simulink model "NPC_1"  (R2013a)
settings: Solver=FixedStepDiscrete  SolverMode=SingleTasking  StartTime=0.0  StopTime=1  FixedStep=Ts  MaxStep=100e-6  MinStep=50e-6  RelTol=1e-3
InitFcn:
  | Ts = 1e-6
libraries: powerlib x72, simulink x6, powerlib_meascontrol x3
settings Model: Creator=Daniel  LastModifiedBy=Daniel
settings SolverCC: InitialStep=50e-6  MaxConsecutiveMinStep=100000  AlgebraicLoopSolver=LineSearch
settings DebuggingCC: ArrayBoundsChecking=warning  AlgebraicLoopMsg=none  ArtificialAlgebraicLoopMsg=none  ParameterPrecisionLossMsg=none  UnconnectedInputMsg=none  UnconnectedOutputMsg=none  UnconnectedLineMsg=none

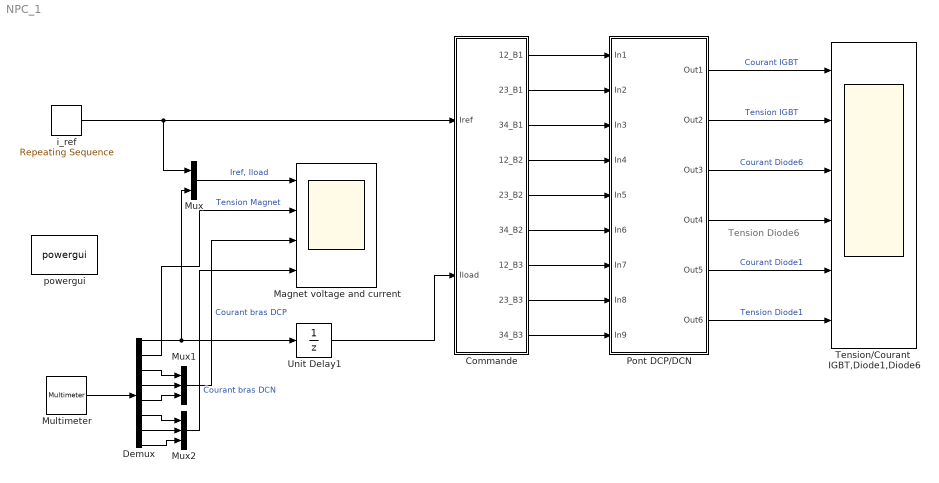
== system NPC_1 ==
  note: Tension Diode6
  Commande : Subsystem  SystemSampleTime=Ts
      settings: MinAlgLoopOccurrences=on
  Demux : Demux  Outputs=8
  Magnet voltage and current : Scope  NumInputPorts=4
      settings: YMin=970~-1000~-12500~-12500  YMax=1030~5000~12500~12500
  Multimeter : powerlib/Measurements/Multimeter  PhasorSimulation=off  OutputType=Complex  sel=[2 1 3 4 5 6 7 8]  L=8  Gain=[1 1 1 1 1 1 1 1]  yselected={'Ib: Pont DCP//DCN/Magnet','Ub: Pont DCP//DCN/Magnet','Ib: Pont DCP//DCN/DC2_B1','Ib: Pont DCP//DCN/DC1_B1','Ib: Pont DCP//DCN/DC1_B2','Ib: Pont DCP//DCN/DC1_B3','Ib: Pont DCP//DCN/DC2_B2','Ib: Pont DCP//DCN/DC2_B3'};  PSBOutputType=1  PSBequivalent=0  AxesSetting=[0,0.1,-100,100]  Display=0  SavedBlockNames=-11
  Mux : Mux  Inputs=2
  Mux1 : Mux  Inputs=3
  Mux2 : Mux  Inputs=3
  Pont DCP/DCN : Subsystem  SystemSampleTime=Ts
      settings: MinAlgLoopOccurrences=on
  Tension/Courant  IGBT,Diode1,Diode6 : Scope  NumInputPorts=6
      settings: YMin=0~-500~0~-2500~-1~-2750  YMax=17500~2500~2000~500~1~0  SaveName=ScopeData2
  Unit Delay1 : UnitDelay  SampleTime=-1
  "i_ref " : simulink/Sources/Repeating Sequence  rep_seq_t=[0 100e-3 475e-3 550e-3 675e-3 900e-3]  rep_seq_y=[0 250 6000 6000 250 250]
  powergui : powerlib/powergui  Priority=1  SimulationMode=Discrete  SolverType=Tustin  SampleTime=Ts  frequency=60  SPID=off  DisableSnubberDevices=off  DisableRonSwitches=off  DisableVfSwitches=off  SwTol=0  Interpol=off  DisplayEquations=off  frequencyindice=0  Pbase=100e6  ErrMax=1e-4  Iterations=50  UnitsV=kV  UnitsW=MW  FunctionMessages=off  echomessages=off  HookPort=off  EnableUseOfTLC=off  x0status=blocks  RestoreLinks=warning  ResistiveCurrentMeasurement=off  Frange=[0:2:500]  Ylog=off  Xlog=on  ShowGrid=off  save=off  variable=ZData  ZoomFFT=off  StartTime=0.0  cycles=1  DisplayStyle=1  fundamental=60  FreqAxis=off  MaxFrequency=1000  frequencyindicesteady=1  RmsSteady=1  display=off  Ts=0  methode=off
  wires:
  Mux/1 -> Magnet voltage and current/1  "Iref, Iload"
  Multimeter/1 -> Demux/1
  Demux/1 -> Unit Delay1/1, Mux/2
  Demux/2 -> Magnet voltage and current/2  "Tension Magnet"
  Demux/3 -> Mux1/1
  Demux/4 -> Mux1/2
  Demux/5 -> Mux1/3
  Demux/6 -> Mux2/1
  Demux/7 -> Mux2/2
  Demux/8 -> Mux2/3
  Mux1/1 -> Magnet voltage and current/3  "Courant bras DCP"
  Mux2/1 -> Magnet voltage and current/4  "Courant bras DCN"
  Pont DCP/DCN/1(Out1) -> Tension/Courant  IGBT,Diode1,Diode6/1  "Courant IGBT"
  Pont DCP/DCN/2(Out2) -> Tension/Courant  IGBT,Diode1,Diode6/2  "Tension IGBT"
  Pont DCP/DCN/3(Out3) -> Tension/Courant  IGBT,Diode1,Diode6/3  "Courant Diode6"
  Pont DCP/DCN/4(Out4) -> Tension/Courant  IGBT,Diode1,Diode6/4
  Pont DCP/DCN/5(Out5) -> Tension/Courant  IGBT,Diode1,Diode6/5  "Courant Diode1"
  Pont DCP/DCN/6(Out6) -> Tension/Courant  IGBT,Diode1,Diode6/6  "Tension Diode1"
  Commande/1(12_B1) -> Pont DCP/DCN/1(In1)
  Commande/2(23_B1) -> Pont DCP/DCN/2(In2)
  Commande/3(34_B1) -> Pont DCP/DCN/3(In3)
  Commande/4(12_B2) -> Pont DCP/DCN/4(In4)
  Commande/5(23_B2) -> Pont DCP/DCN/5(In5)
  Commande/6("34_B2 ") -> Pont DCP/DCN/6(In6)
  Commande/7(12_B3) -> Pont DCP/DCN/7(In7)
  Commande/8(23_B3) -> Pont DCP/DCN/8(In8)
  Commande/9("34_B3 ") -> Pont DCP/DCN/9(In9)
  "i_ref "/1 -> Commande/1(Iref), Mux/1
  Unit Delay1/1 -> Commande/2("Iload ")

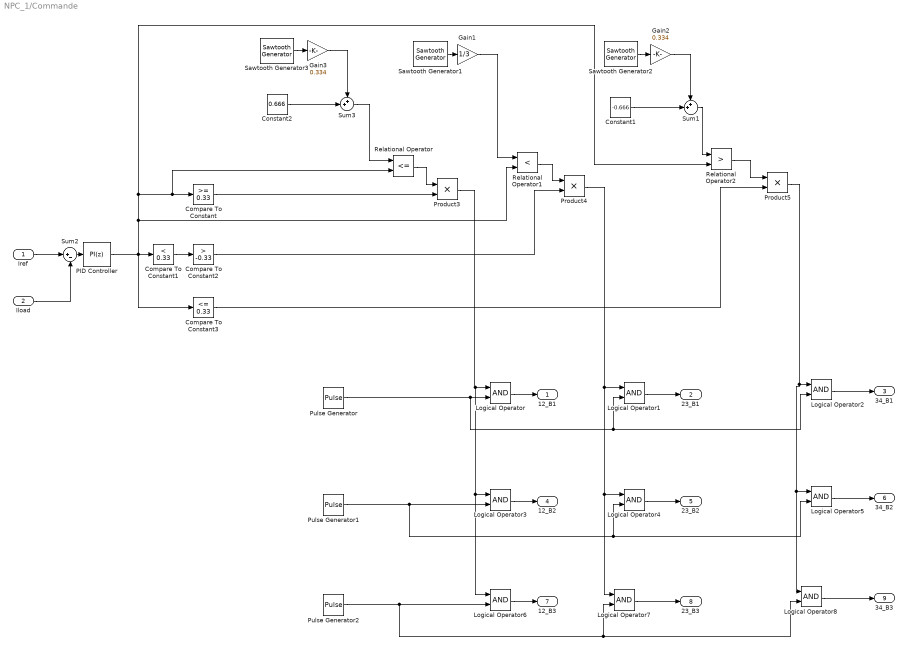
== system NPC_1/Commande ==
  Iref : Inport
  "Iload " : Inport  Port=2
  Compare To Constant : simulink/Logic and Bit Operations/Compare To Constant  relop=>=  const=0.33  OutDataTypeStr=boolean
  Compare To Constant1 : simulink/Logic and Bit Operations/Compare To Constant  relop=<  const=0.33  OutDataTypeStr=boolean
  Compare To Constant2 : simulink/Logic and Bit Operations/Compare To Constant  relop=>  const=-0.33  OutDataTypeStr=boolean
  Compare To Constant3 : simulink/Logic and Bit Operations/Compare To Constant  relop=<=  const=0.33  OutDataTypeStr=boolean
  Constant1 : Constant  Value=-0.666  SampleTime=Ts
  Constant2 : Constant  Value=0.666  SampleTime=Ts
  Gain1 : Gain  Gain=1/3  SampleTime=Ts
  Gain2 : Gain  Gain=0.334  SampleTime=Ts
  Gain3 : Gain  Gain=0.334  SampleTime=Ts
  Logical Operator{,1..8} (9 alike) : Logic  AllPortsSameDT=off  OutDataTypeStr=boolean  SampleTime=Ts
  PID Controller : simulink/Continuous/PID Controller  Controller=PI  TimeDomain=Discrete-time  SampleTime=Ts  IntegratorMethod=Forward Euler  FilterMethod=Forward Euler  Form=Parallel  P=1.05611  I=24.6  D=0  N=100  InitialConditionSource=internal  InitialConditionForIntegrator=0  InitialConditionForFilter=0  ExternalReset=none  LimitOutput=on  UpperSaturationLimit=1  LowerSaturationLimit=-1  LinearizeAsGain=on  AntiWindupMode=clamping  Kb=1  TrackingMode=off  Kt=1  PParamMin=[]  PParamMax=[]  IParamMin=[]  IParamMax=[]  DParamMin=[]  DParamMax=[]  NParamMin=[]  NParamMax=[]  KbParamMin=[]  KbParamMax=[]  KtParamMin=[]  KtParamMax=[]  POutMin=[]  POutMax=[]  IOutMin=[]  IOutMax=[]  DOutMin=[]  DOutMax=[]  NOutMin=[]  NOutMax=[]  KbOutMin=[]  KbOutMax=[]  KtOutMin=[]  KtOutMax=[]  IntegratorOutMin=[]  IntegratorOutMax=[]  FilterOutMin=[]  FilterOutMax=[]  SumOutMin=[]  SumOutMax=[]  SumI1OutMin=[]  SumI1OutMax=[]  SumI2OutMin=[]  SumI2OutMax=[]  SumI3OutMin=[]  SumI3OutMax=[]  SumDOutMin=[]  SumDOutMax=[]  SaturationOutMin=[]  SaturationOutMax=[]  IntegratorContinuousStateAttributes=''  IntegratorStateMustResolveToSignalObject=off  IntegratorRTWStateStorageClass=Auto  FilterContinuousStateAttributes=''  FilterStateMustResolveToSignalObject=off  FilterRTWStateStorageClass=Auto
  Product3 : Product  SampleTime=Ts
  Product4 : Product  SampleTime=Ts
  Product5 : Product  SampleTime=Ts
  Pulse Generator : DiscretePulseGenerator  Period=floor(3e-3/Ts)  PulseWidth=floor(1e-3/Ts)  SampleTime=Ts
  Pulse Generator1 : DiscretePulseGenerator  Period=floor(3e-3/Ts)  PulseWidth=floor(1e-3/Ts)  PhaseDelay=floor(1e-3/Ts)  SampleTime=Ts
  Pulse Generator2 : DiscretePulseGenerator  Period=floor(3e-3/Ts)  PulseWidth=floor(1e-3/Ts)  PhaseDelay=floor(2e-3/Ts)  SampleTime=Ts
  Relational Operator : RelationalOperator  Operator=<=  OutDataTypeStr=boolean  SampleTime=Ts
  Relational Operator1 : RelationalOperator  Operator=<  OutDataTypeStr=boolean  SampleTime=Ts
  Relational Operator2 : RelationalOperator  Operator=>  OutDataTypeStr=boolean  SampleTime=Ts
  Sawtooth Generator1 : powerlib_meascontrol/Pulse & Signal Generators/Sawtooth Generator  Freq=1e3  Phase=0  Ts=Ts
  Sawtooth Generator2 : powerlib_meascontrol/Pulse & Signal Generators/Sawtooth Generator  Freq=1e3  Phase=0  Ts=Ts
  Sawtooth Generator3 : powerlib_meascontrol/Pulse & Signal Generators/Sawtooth Generator  Freq=1e3  Phase=0  Ts=Ts
  Sum1 : Sum  Inputs=++|
  Sum2 : Sum  Inputs=|+-
  Sum3 : Sum  Inputs=++|
  12_B1 : Outport
  23_B1 : Outport  Port=2
  34_B1 : Outport  Port=3
  12_B2 : Outport  Port=4
  23_B2 : Outport  Port=5
  "34_B2 " : Outport  Port=6
  12_B3 : Outport  Port=7
  23_B3 : Outport  Port=8
  "34_B3 " : Outport  Port=9
  wires:
  Constant1/1 -> Sum1/2
  Sawtooth Generator1/1 -> Gain1/1
  Gain2/1 -> Sum1/1
  Sawtooth Generator2/1 -> Gain2/1
  Iref/1 -> Sum2/1
  "Iload "/1 -> Sum2/2
  Sum2/1 -> PID Controller/1
  Compare To Constant1/1 -> Compare To Constant2/1
  Compare To Constant/1 -> Product3/2
  Compare To Constant2/1 -> Product4/2
  Compare To Constant3/1 -> Product5/2
  PID Controller/1 -> Relational Operator2/2, Relational Operator/2, Compare To Constant/1, Relational Operator1/2, Compare To Constant3/1, Compare To Constant1/1
  Gain1/1 -> Relational Operator1/1
  Sum1/1 -> Relational Operator2/1
  Pulse Generator/1 -> Logical Operator2/2, Logical Operator1/2, Logical Operator/2
  Pulse Generator1/1 -> Logical Operator3/2, Logical Operator5/2, Logical Operator4/2
  Pulse Generator2/1 -> Logical Operator8/2, Logical Operator7/2, Logical Operator6/2
  Logical Operator/1 -> 12_B1/1
  Logical Operator1/1 -> 23_B1/1
  Logical Operator2/1 -> 34_B1/1
  Logical Operator4/1 -> 23_B2/1
  Logical Operator7/1 -> 23_B3/1
  Logical Operator3/1 -> 12_B2/1
  Logical Operator6/1 -> 12_B3/1
  Logical Operator5/1 -> "34_B2 "/1
  Logical Operator8/1 -> "34_B3 "/1
  Sum3/1 -> Relational Operator/1
  Relational Operator/1 -> Product3/1
  Product3/1 -> Logical Operator6/1, Logical Operator3/1, Logical Operator/1
  Relational Operator1/1 -> Product4/1
  Product4/1 -> Logical Operator7/1, Logical Operator4/1, Logical Operator1/1
  Relational Operator2/1 -> Product5/1
  Product5/1 -> Logical Operator8/1, Logical Operator5/1, Logical Operator2/1
  Constant2/1 -> Sum3/2
  Gain3/1 -> Sum3/1
  Sawtooth Generator3/1 -> Gain3/1

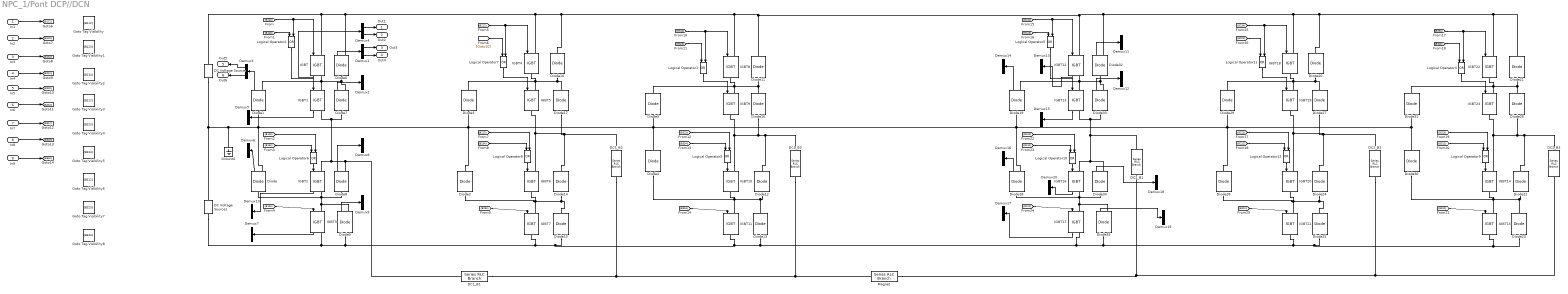
== system NPC_1/Pont DCP//DCN ==
  In1 : Inport
  In2 : Inport  Port=2
  In3 : Inport  Port=3
  In4 : Inport  Port=4
  In5 : Inport  Port=5
  In6 : Inport  Port=6
  In7 : Inport  Port=7
  In8 : Inport  Port=8
  In9 : Inport  Port=9
  DC Voltage Source : powerlib/Electrical Sources/DC Voltage Source  Amplitude=2500  Measurements=None
  DC Voltage Source1 : powerlib/Electrical Sources/DC Voltage Source  Amplitude=2500  Measurements=None
  DC1_B1 : powerlib/Elements/Series RLC Branch  LConnTagsString=__new0  RConnTagsString=__new0  BranchType=L  Resistance=0  Inductance=1e-6  SetiL0=off  InitialCurrent=0  Capacitance=1e-6  Setx0=off  InitialVoltage=0  Measurements=Branch current
  DC1_B2 : powerlib/Elements/Series RLC Branch  LConnTagsString=__new0  RConnTagsString=__new0  BranchType=L  Resistance=0  Inductance=1e-6  SetiL0=off  InitialCurrent=0  Capacitance=1e-6  Setx0=off  InitialVoltage=0  Measurements=Branch current
  DC1_B3 : powerlib/Elements/Series RLC Branch  LConnTagsString=__new0  RConnTagsString=__new0  BranchType=L  Resistance=0  Inductance=1e-6  SetiL0=off  InitialCurrent=0  Capacitance=1e-6  Setx0=off  InitialVoltage=0  Measurements=Branch current
  DC2_B1 : powerlib/Elements/Series RLC Branch  LConnTagsString=__new0  RConnTagsString=__new0  BranchType=L  Resistance=0  Inductance=1e-6  SetiL0=off  InitialCurrent=0  Capacitance=1e-6  Setx0=off  InitialVoltage=0  Measurements=Branch current
  DC2_B2 : powerlib/Elements/Series RLC Branch  LConnTagsString=__new0  RConnTagsString=__new0  BranchType=L  Resistance=0  Inductance=1e-6  SetiL0=off  InitialCurrent=0  Capacitance=1e-6  Setx0=off  InitialVoltage=0  Measurements=Branch current
  DC2_B3 : powerlib/Elements/Series RLC Branch  LConnTagsString=__new0  RConnTagsString=__new0  BranchType=L  Resistance=0  Inductance=1e-6  SetiL0=off  InitialCurrent=0  Capacitance=1e-6  Setx0=off  InitialVoltage=0  Measurements=Branch current
  Demux{1..20} (20 alike) : Demux  Outputs=2
  Diode{,1,6..9,18..19,32..35} (12 alike) : powerlib/Power Electronics/Diode  Ron=0.001  Lon=0  Vf=0.8  IC=0  UseSnubber=off  Rs=1  Cs=inf  Measurements=on
  Diode{2..5,10..17,20..31} (24 alike) : powerlib/Power Electronics/Diode  Ron=0.001  Lon=0  Vf=0.8  IC=0  UseSnubber=off  Rs=1  Cs=inf  Measurements=off
  Goto Tag Visibility : GotoTagVisibility  GotoTag=B112
  Goto Tag Visibility1 : GotoTagVisibility  GotoTag=B123
  Goto Tag Visibility2 : GotoTagVisibility  GotoTag=B134
  Goto Tag Visibility3 : GotoTagVisibility  GotoTag=B212
  Goto Tag Visibility4 : GotoTagVisibility  GotoTag=B223
  Goto Tag Visibility5 : GotoTagVisibility  GotoTag=B234
  Goto Tag Visibility6 : GotoTagVisibility  GotoTag=B312
  Goto Tag Visibility7 : GotoTagVisibility  GotoTag=B323
  Goto Tag Visibility8 : GotoTagVisibility  GotoTag=B334
  Ground2 : powerlib/Elements/Ground  LConnTagsString=a
  IGBT{,1..3,12..13,16..17} (8 alike) : powerlib/Power Electronics/IGBT  Ron=0.001  Lon=0  Vf=1  Tf=1e-6  Tt=2e-6  IC=0  Rs=0  Cs=0  Measurements=on
  IGBT{4..11,14..15,18..23} (16 alike) : powerlib/Power Electronics/IGBT  Ron=0.001  Lon=0  Vf=1  Tf=1e-6  Tt=2e-6  IC=0  Rs=0  Cs=0  Measurements=off
  Logical Operator{1..12} (12 alike) : Logic  Operator=OR  AllPortsSameDT=off  OutDataTypeStr=boolean
  Magnet : powerlib/Elements/Series RLC Branch  LConnTagsString=__new0  RConnTagsString=__new0  BranchType=RL  Resistance=0.28  Inductance=0.1  SetiL0=off  InitialCurrent=0  Capacitance=1e-6  Setx0=off  InitialVoltage=0  Measurements=Branch voltage and current
  Out1 : Outport
  Out2 : Outport  Port=2
  Out3 : Outport  Port=3
  Out4 : Outport  Port=4
  Out5 : Outport  Port=5
  Out6 : Outport  Port=6
  tag scope: B112=scoped, B123=scoped, B134=scoped, B212=scoped, B223=scoped, B234=scoped, B312=scoped, B323=scoped, B334=scoped
  wires:
  IGBT12/1 -> Demux13/1
  Diode34/1 -> Demux18/1
  Diode35/1 -> Demux19/1
  Logical Operator7/1 -> IGBT5/1
  Diode7/1 -> Demux2/1
  Logical Operator3/1 -> IGBT10/1
  Logical Operator1/1 -> IGBT9/1
  [B323] -> Logical Operator3/2
  [B334] -> Logical Operator3/1
  [B123] -> Logical Operator10/2
  Diode18/1 -> Demux16/1
  Logical Operator10/1 -> IGBT16/1
  [B223] -> Logical Operator12/2
  [B112] -> IGBT17/1
  [B212] -> IGBT21/1
  [B123] -> Logical Operator5/1
  [B112] -> Logical Operator10/1
  [B212] -> Logical Operator12/1
  Logical Operator6/1 -> IGBT2/1
  [B223] -> Logical Operator8/2
  [B112] -> IGBT/1, Logical Operator2/2
  [B323] -> Logical Operator1/1
  [B234] -> Logical Operator8/1
  Diode1/1 -> Demux3/1
  [B234] -> Logical Operator11/2, IGBT18/1
  [B334] -> IGBT22/1, Logical Operator4/2
  Logical Operator12/1 -> IGBT20/1
  [B323] -> Logical Operator9/2
  [B312] -> IGBT15/1
  Logical Operator4/1 -> IGBT23/1
  [B223] -> Logical Operator11/1
  Logical Operator5/1 -> IGBT13/1
  Logical Operator11/1 -> IGBT19/1
  Logical Operator9/1 -> IGBT14/1
  [B212] -> Logical Operator7/2, IGBT4/1
  Logical Operator2/1 -> IGBT1/1
  IGBT16/1 -> Demux20/1
  [B134] -> IGBT3/1
  [B323] -> Logical Operator4/1
  [B134] -> IGBT12/1, Logical Operator5/2
  Diode9/1 -> Demux9/1
  [B123] -> Logical Operator6/2
  [B134] -> Logical Operator6/1
  [B123] -> Logical Operator2/1
  [B312] -> IGBT8/1, Logical Operator1/2
  [B334] -> IGBT11/1
  [B234] -> IGBT7/1
  [B312] -> Logical Operator9/1
  [Goto10] -> Logical Operator7/1
  Diode8/1 -> Demux8/1
  Diode19/1 -> Demux14/1
  IGBT3/1 -> Demux7/1
  Diode6/1 -> Demux1/1
  Diode/1 -> Demux6/1
  IGBT/1 -> Demux4/1
  IGBT17/1 -> Demux17/1
  IGBT1/1 -> Demux5/1
  Logical Operator8/1 -> IGBT6/1
  Diode33/1 -> Demux12/1
  IGBT2/1 -> Demux10/1
  IGBT13/1 -> Demux15/1
  Diode32/1 -> Demux11/1
  In1/1 -> [B112]
  In2/1 -> [B123]
  In3/1 -> [B134]
  In4/1 -> [B212]
  In5/1 -> [B223]
  In6/1 -> [B234]
  In7/1 -> [B312]
  In8/1 -> [B323]
  In9/1 -> [B334]
  Demux4/1 -> Out1/1
  Demux4/2 -> Out2/1
  Demux1/1 -> Out3/1
  Demux1/2 -> Out4/1
  Demux3/1 -> Out5/1
  Demux3/2 -> Out6/1
  connections:
  IGBT5/RConn1 -- IGBT6/LConn1 -- DC1_B2/LConn1 -- Diode14/RConn1 -- Diode17/LConn1
  IGBT8/RConn1 -- Diode5/RConn1 -- Diode11/LConn1 -- Diode16/RConn1 -- IGBT9/LConn1
  IGBT18/RConn1 -- Diode29/RConn1 -- IGBT19/LConn1 -- Diode27/RConn1 -- Diode20/LConn1
  Diode12/LConn1 -- Diode13/RConn1 -- Diode4/LConn1 -- IGBT10/RConn1 -- IGBT11/LConn1
  IGBT4/RConn1 -- Diode3/RConn1 -- Diode17/RConn1 -- Diode10/LConn1 -- IGBT5/LConn1
  IGBT2/RConn1 -- Diode/LConn1 -- IGBT3/LConn1 -- Diode9/RConn1 -- Diode8/LConn1
  IGBT10/LConn1 -- IGBT9/RConn1 -- Diode16/LConn1 -- Diode12/RConn1 -- DC1_B3/LConn1
  Diode19/LConn1 -- Diode4/RConn1 -- Diode5/LConn1 -- Diode2/RConn1 -- Diode3/LConn1 -- DC Voltage Source1/RConn1 -- DC Voltage Source/LConn1 -- Ground2/LConn1 -- Diode/RConn1 -- Diode1/LConn1 -- Diode18/RConn1 -- Diode28/RConn1 -- Diode29/LConn1 -- Diode30/RConn1 -- Diode31/LConn1
  IGBT1/RConn1 -- Diode7/LConn1 -- DC1_B1/LConn1 -- Diode8/RConn1 -- IGBT2/LConn1
  IGBT15/LConn1 -- Diode30/LConn1 -- IGBT14/RConn1 -- Diode23/RConn1 -- Diode22/LConn1
  IGBT13/RConn1 -- DC2_B1/LConn1 -- Diode34/RConn1 -- IGBT16/LConn1 -- Diode33/LConn1
  Diode32/RConn1 -- Diode11/RConn1 -- IGBT8/LConn1 -- Diode10/RConn1 -- IGBT4/LConn1 -- IGBT/LConn1 -- DC Voltage Source/RConn1 -- Diode6/RConn1 -- IGBT12/LConn1 -- IGBT18/LConn1 -- Diode20/RConn1 -- IGBT22/LConn1 -- Diode21/RConn1
  IGBT16/RConn1 -- Diode18/LConn1 -- Diode34/LConn1 -- IGBT17/LConn1 -- Diode35/RConn1
  DC2_B2/RConn1 -- DC2_B3/RConn1 -- Magnet/RConn1 -- DC2_B1/RConn1
  IGBT22/RConn1 -- Diode31/RConn1 -- Diode21/LConn1 -- Diode26/RConn1 -- IGBT23/LConn1
  IGBT/RConn1 -- Diode1/RConn1 -- Diode7/RConn1 -- Diode6/LConn1 -- IGBT1/LConn1
  IGBT6/RConn1 -- Diode15/RConn1 -- Diode14/LConn1 -- Diode2/LConn1 -- IGBT7/LConn1
  IGBT19/RConn1 -- IGBT20/LConn1 -- DC2_B2/LConn1 -- Diode24/RConn1 -- Diode27/LConn1
  IGBT20/RConn1 -- Diode25/RConn1 -- Diode24/LConn1 -- Diode28/LConn1 -- IGBT21/LConn1
  IGBT7/RConn1 -- Diode13/LConn1 -- Diode35/LConn1 -- IGBT21/RConn1 -- Diode25/LConn1 -- IGBT15/RConn1 -- Diode23/LConn1 -- IGBT17/RConn1 -- IGBT11/RConn1 -- Diode15/LConn1 -- DC Voltage Source1/LConn1 -- IGBT3/RConn1 -- Diode9/LConn1
  DC2_B3/LConn1 -- Diode22/RConn1 -- Diode26/LConn1 -- IGBT23/RConn1 -- IGBT14/LConn1
  DC1_B3/RConn1 -- Magnet/LConn1 -- DC1_B2/RConn1 -- DC1_B1/RConn1
  IGBT12/RConn1 -- Diode19/RConn1 -- IGBT13/LConn1 -- Diode33/RConn1 -- Diode32/LConn1
